simulink model "TestSimulinkNoise"  (R2022a)
settings: Solver=VariableStepAuto  StartTime=0.0  StopTime=10  RelTol=1e-3
model workspace (MAT data in the model file):
  Q = [0.4; 1000]
settings Model: Creator=tyevans  LastModifiedBy=tyevans

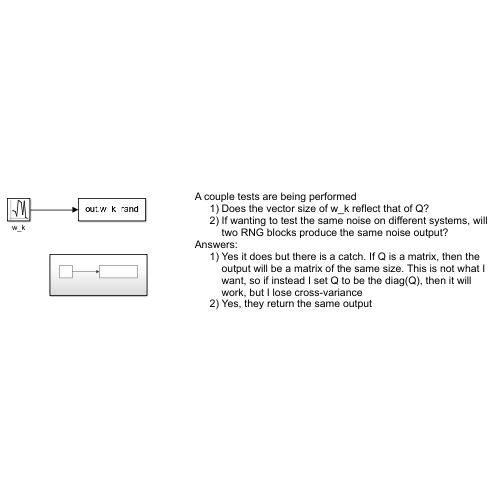
[thumbnail: Simulink's stored preview of the top-level diagram]
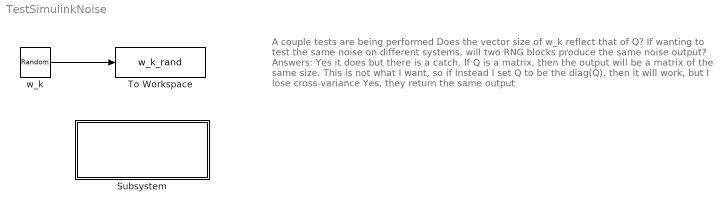
== system TestSimulinkNoise ==
  note: A couple tests are being performed
      | Does the vector size of w_k reflect that of Q?
      | If wanting to test the same noise on different systems, will two RNG blocks produce the same noise output?
      | Answers:
      | Yes it does but there is a catch. If Q is a matrix, then the output will be a matrix of the same size. This is not what I want, so if instead I set Q to be the diag(Q), then it will work, but I lose cross-variance
      | Yes, they return the same output
  Subsystem : Subsystem
  To Workspace : ToWorkspace  VariableName=w_k_rand  SampleTime=-1
  w_k : RandomNumber  Variance=Q  Seed=1  SampleTime=1  VectorParams1D=off
  wires:
  w_k/1 -> To Workspace/1

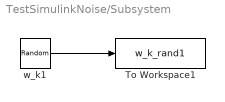
== system TestSimulinkNoise/Subsystem ==
  To Workspace1 : ToWorkspace  VariableName=w_k_rand1  SampleTime=-1
  w_k1 : RandomNumber  Variance=Q  Seed=1  SampleTime=1  VectorParams1D=off
  wires:
  w_k1/1 -> To Workspace1/1
